simulink model "chemical_calculator"  (R2019a)
settings: Solver=VariableStepAuto  StartTime=0.0  StopTime=15  RelTol=1e-3
settings Model: Creator=ricka  LastModifiedBy=ricka

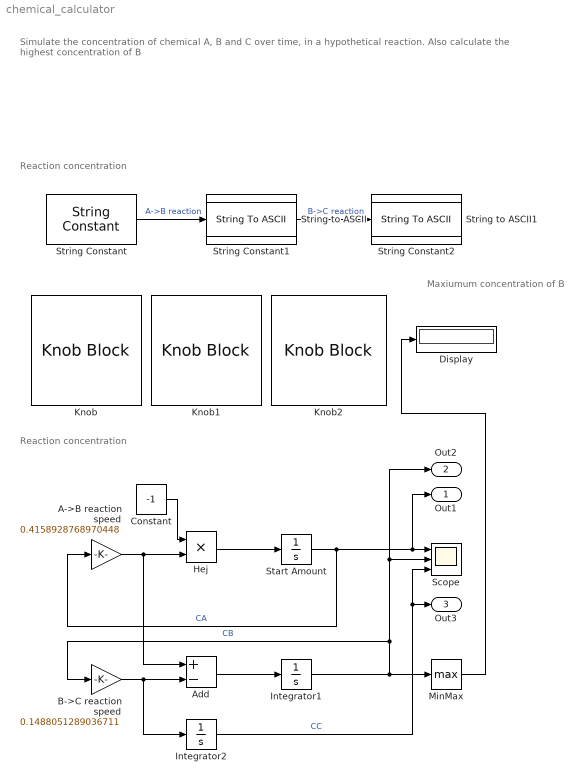
== system chemical_calculator ==
  note: Maxiumum
      | concentration
      | of B
  note: Reaction concentration
  note: Reaction concentration
  note: Simulate the concentration of chemical A, B and C over time, in a hypothetical reaction.
      | Also calculate the highest concentration of B
  "A->B reaction speed " : Gain  Gain=0.4158928768970448
  Add : Sum  Inputs=+-
  "B->C reaction speed " : Gain  Gain=0.1488051289036711
  Constant : Constant  Value=-1
  Display : Display
  "Hej " : Product
  Integrator1 : Integrator
  Integrator2 : Integrator
  Knob : KnobBlock  Description=Hello  ScaleMax=2
  Knob1 : KnobBlock  ScaleMax=2
  Knob2 : KnobBlock  ScaleMax=20
  MinMax : MinMax  Function=max
  Scope : Scope  NumInputPorts=3
  "Start Amount " : Integrator  InitialCondition=4.288551802460194
  String Constant : StringConstant  String="\"Chemical A'\""
  String Constant1 : StringConstant  String="\"Chemical B'\""
  String Constant2 : StringConstant  String="\"Chemical C\""
  String to ASCII : StringToASCII
  String to ASCII1 : StringToASCII
  Out1 : Outport
  Out2 : Outport  Port=2
  Out3 : Outport  Port=3
  wires:
  "A->B reaction speed "/1 -> Add/1, "Hej "/2
  Constant/1 -> "Hej "/1
  "Hej "/1 -> "Start Amount "/1
  "Start Amount "/1 -> "A->B reaction speed "/1, Out1/1, Scope/1  "CA"
  "B->C reaction speed "/1 -> Integrator2/1, Add/2
  Add/1 -> Integrator1/1
  Integrator1/1 -> MinMax/1, "B->C reaction speed "/1, Scope/2, Out2/1  "CB"
  Integrator2/1 -> Scope/3, Out3/1  "CC"
  String Constant/1 -> String to ASCII/1  "A->B reaction"
  String Constant1/1 -> String to ASCII1/1  "B->C reaction"
  MinMax/1 -> Display/1
